simulink model "ControlerFuzzy"  (R2016a)
settings: Solver=ode5  StartTime=0.0  StopTime=600  FixedStep=0.1  RelTol=1e-3
libraries: fuzblock x1
settings Model: Creator=Andrada  LastModifiedBy=Andrada
settings DataIOCC: SignalLoggingName=sigout

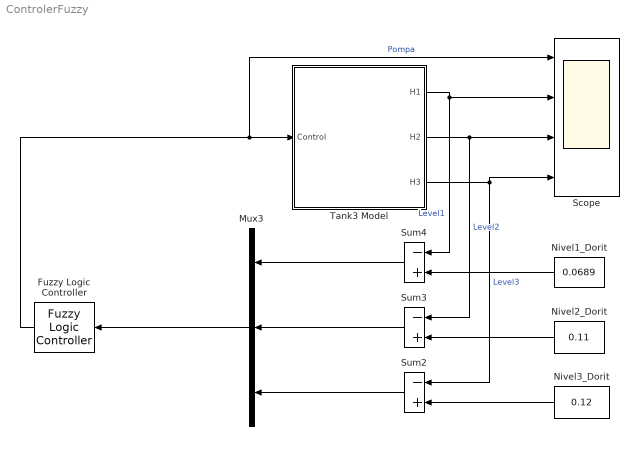
== system ControlerFuzzy ==
  Fuzzy Logic Controller : fuzblock/Fuzzy Logic  Controller  fis='controlerMultitank.fis'
  Mux3 : Mux  Inputs=3
  Nivel1_Dorit : Constant  Value=0.0689
  Nivel2_Dorit : Constant  Value=0.11
  Nivel3_Dorit : Constant  Value=0.12
  Scope : Scope  NumInputPorts=4
  Sum2 : Sum  Inputs=-+  SaturateOnIntegerOverflow=on  InputSameDT=on  OutDataTypeStr=Inherit: Same as first input
  Sum3 : Sum  Inputs=-+  SaturateOnIntegerOverflow=on  InputSameDT=on  OutDataTypeStr=Inherit: Same as first input
  Sum4 : Sum  Inputs=-+  SaturateOnIntegerOverflow=on  InputSameDT=on  OutDataTypeStr=Inherit: Same as first input
  Tank3 Model : Subsystem  mask{H0=[ 0.001 0.001 0.001 ], C=[11.08 8.43 8.28] * 1E-5, Alfa=[ 0.5 0.5 0.5 ], UT=[ 0.25 0.035 ], MT=[ 0.348 0.1 0.35 ], LT=[ 0.365 0.35 ]}
      mask prompts: H0 "Initial Conditions [ H10 H20 H30 ]:"; C "[ C1 C2 C3 ]:"; Alfa "[ Alfa1 Alfa2 Alfa3 ]:"; UT "Upper Tank [ a w ]:"; MT "Middle Tank [ b c H2max ]:"; LT "Lower Tank [ R H3max ]:"
      mask init:
      | C1=C(1); C2=C(2); C3=C(3);
      | Alfa1 = Alfa(1); Alfa2 = Alfa(2); Alfa3 = Alfa(3); 
      | a = UT(1); w = UT(2);
      | b = MT(1); c = MT(2); H2max = MT(3);
      | R = LT(1); H3max = LT(2);
      mask Display: plot([0.1 0.9 0.9 0.1 0.1], [ 0 0 1 1 0], [0.2 0.8 0.8 0.2 0.2], [0.05 0.05 0.2 0.2 0.05], [0.4 0.65 0.72 0.72 0.4], [0.7 0.5 0.5 0.7 0.7], [ 0.4 0.5000 0.5200 0.5397 0.5591 0.5779 0.5959 0.6129 0.6288 0.6435 0.6567 0.6683 0.6782 0.6864 0.6927 0.6971 0.6995 0.7 0.4 0.4 ], [0.25 0.2500 0.2510 0.2540 0.2589 0.2658 0.2745 0.2849 0.2970 0.3107 0.3257 0.3419 0.3593 0.3775 0.3965 0.4160 0.4359 0.45 0.45 0.25], [0.3 0.55 0.55 0.3 0.3], [0.75 0.75 0.95 0.95 0.75] )
  wires:
  Tank3 Model/1(H1) -> Scope/2, Sum4/1  "Level1"
  Tank3 Model/2(H2) -> Scope/3, Sum3/1  "Level2"
  Tank3 Model/3(H3) -> Scope/4, Sum2/1  "Level3"
  Nivel1_Dorit/1 -> Sum4/2
  Nivel2_Dorit/1 -> Sum3/2
  Nivel3_Dorit/1 -> Sum2/2
  Fuzzy Logic Controller/1 -> Scope/1, Tank3 Model/1(Control)  "Pompa"
  Sum3/1 -> Mux3/2
  Sum2/1 -> Mux3/3
  Mux3/1 -> Fuzzy Logic Controller/1
  Sum4/1 -> Mux3/1

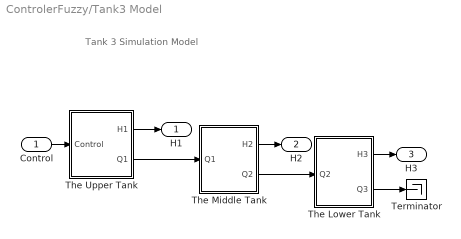
== system ControlerFuzzy/Tank3 Model ==
  note: Tank 3 Simulation Model
  Control : Inport
  Terminator : Terminator
  The Lower Tank : Subsystem
  The Middle Tank : Subsystem
  The Upper Tank : Subsystem
  H1 : Outport
  H2 : Outport  Port=2
  H3 : Outport  Port=3
  wires:
  The Upper Tank/2(Q1) -> The Middle Tank/1(Q1)
  The Middle Tank/2(Q2) -> The Lower Tank/1(Q2)
  The Upper Tank/1(H1) -> H1/1
  The Middle Tank/1(H2) -> H2/1
  Control/1 -> The Upper Tank/1(Control)
  The Lower Tank/1(H3) -> H3/1
  The Lower Tank/2(Q3) -> Terminator/1

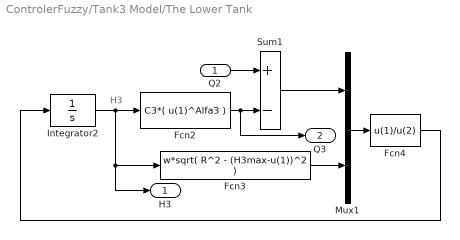
== system ControlerFuzzy/Tank3 Model/The Lower Tank ==
  note: H3
  Q2 : Inport
  Fcn2 : Fcn  Expr=C3*( u(1)^Alfa3 )
  Fcn3 : Fcn  Expr=w*sqrt( R^2 - (H3max-u(1))^2 )
  Fcn4 : Fcn  Expr=u(1)/u(2)
  Integrator2 : Integrator  InitialCondition=H0(3)  LimitOutput=on  UpperSaturationLimit=0.3  LowerSaturationLimit=0.001
  Mux1 : Mux  Inputs=2
  Sum1 : Sum  Inputs=+-  SaturateOnIntegerOverflow=on  InputSameDT=on  OutDataTypeStr=Inherit: Same as first input
  H3 : Outport
  Q3 : Outport  Port=2
  wires:
  Integrator2/1 -> Fcn2/1, Fcn3/1, H3/1
  Fcn3/1 -> Mux1/2
  Fcn4/1 -> Integrator2/1
  Sum1/1 -> Mux1/1
  Fcn2/1 -> Sum1/2, Q3/1
  Q2/1 -> Sum1/1
  Mux1/1 -> Fcn4/1

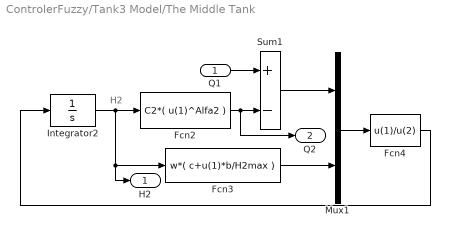
== system ControlerFuzzy/Tank3 Model/The Middle Tank ==
  note: H2
  Q1 : Inport
  Fcn2 : Fcn  Expr=C2*( u(1)^Alfa2 )
  Fcn3 : Fcn  Expr=w*( c+u(1)*b/H2max )
  Fcn4 : Fcn  Expr=u(1)/u(2)
  Integrator2 : Integrator  InitialCondition=H0(2)  LimitOutput=on  UpperSaturationLimit=0.3  LowerSaturationLimit=0.001
  Mux1 : Mux  Inputs=2
  Sum1 : Sum  Inputs=+-  SaturateOnIntegerOverflow=on  InputSameDT=on  OutDataTypeStr=Inherit: Same as first input
  H2 : Outport
  Q2 : Outport  Port=2
  wires:
  Mux1/1 -> Fcn4/1
  Q1/1 -> Sum1/1
  Fcn2/1 -> Q2/1, Sum1/2
  Sum1/1 -> Mux1/1
  Fcn4/1 -> Integrator2/1
  Fcn3/1 -> Mux1/2
  Integrator2/1 -> H2/1, Fcn3/1, Fcn2/1

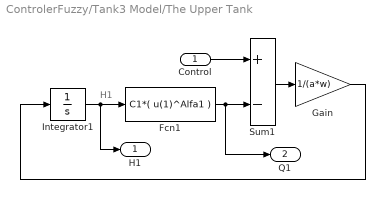
== system ControlerFuzzy/Tank3 Model/The Upper Tank ==
  note: H1
  Control : Inport
  Fcn1 : Fcn  Expr=C1*( u(1)^Alfa1 )
  Gain : Gain  Gain=1/(a*w)  SaturateOnIntegerOverflow=on  OutDataTypeStr=Inherit: Same as input  ParamDataTypeStr=Inherit: Same as input
  Integrator1 : Integrator  InitialCondition=H0(1)  LimitOutput=on  UpperSaturationLimit=0.3  LowerSaturationLimit=0.001
  Sum1 : Sum  Inputs=+-  SaturateOnIntegerOverflow=on  InputSameDT=on  OutDataTypeStr=Inherit: Same as first input
  H1 : Outport
  Q1 : Outport  Port=2
  wires:
  Gain/1 -> Integrator1/1
  Sum1/1 -> Gain/1
  Fcn1/1 -> Sum1/2, Q1/1
  Control/1 -> Sum1/1
  Integrator1/1 -> H1/1, Fcn1/1
